simulink model "tesla_model"  (R2017b)
settings: Solver=VariableStepAuto  StartTime=0.0  StopTime=time  RelTol=1e-3
values from neighbouring files (symbols this model uses):
  fd = 0.5*density*A*C_D    (= 0.34398)    [tesla_model.m]
  fr = mass*g*C_r    (= 413.5896)    [tesla_model.m]
  ft = G_r*eta*(1/r)    (= 28.3791666667)    [tesla_model.m]
  G_r = 9.73    [tesla_model.m]
  K_E = 0.12    [tesla_model.m]
  K_T = 0.25    [tesla_model.m]
  L = 493*10^(-9)    (= 4.93e-07)    [tesla_model.m]
  lowLimit = 0    [tesla_model.m]
  mass = 2108    [tesla_model.m]
  r = 0.5*d    (= 0.24)    [tesla_model.m]
  R = 5.3*10^(-3)    (= 0.0053)    [tesla_model.m]
  uppLimit = 601    [tesla_model.m]
  V = mod*groups*v_nom    (= 345.6)    [tesla_model.m]
settings Model: Creator=User1  LastModifiedBy=User1

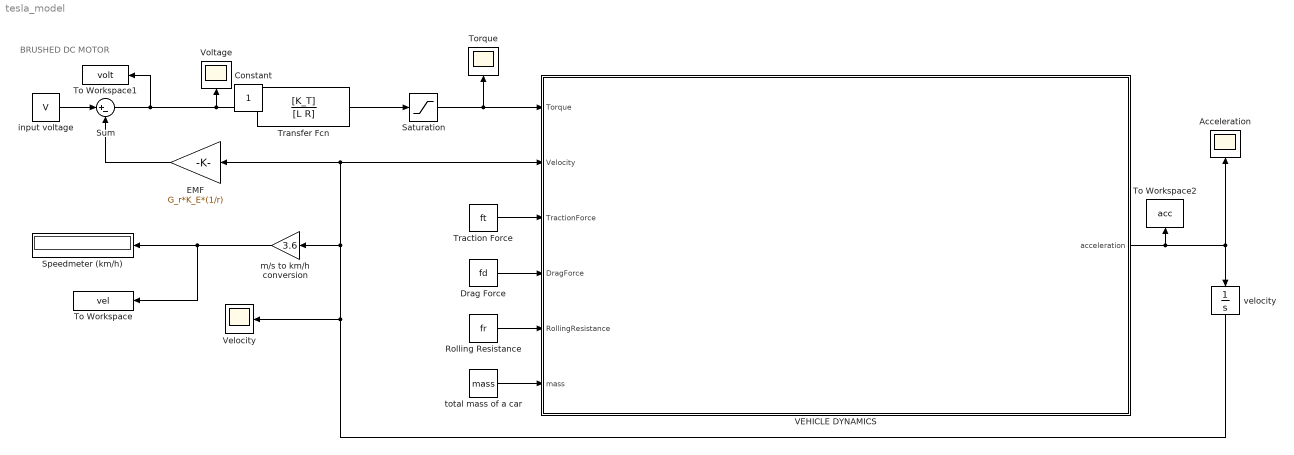
== system tesla_model ==
  note: BRUSHED DC MOTOR
  Acceleration : Scope
  Drag Force : Constant  Value=fd
  EMF : Gain  Gain=G_r*K_E*(1/r)
  Rolling Resistance : Constant  Value=fr
  Saturation : Saturate  UpperLimit=uppLimit  LowerLimit=lowLimit
  Speedmeter (km/h) : Display
  Sum : Sum  Inputs=|+-
  To Workspace : ToWorkspace  VariableName=vel  SaveFormat=Timeseries  SampleTime=-1
      settings: Save2DSignal=2-D array (concatenate along first dimension)
  To Workspace1 : ToWorkspace  VariableName=volt  SaveFormat=Timeseries  SampleTime=-1
      settings: Save2DSignal=2-D array (concatenate along first dimension)
  To Workspace2 : ToWorkspace  VariableName=acc  SaveFormat=Timeseries  SampleTime=-1
  Torque : Scope
  Traction Force : Constant  Value=ft
  Transfer Fcn : TransferFcn  Numerator=[K_T]  Denominator=[L R]
  VEHICLE DYNAMICS : MATLAB Function  TreatAsAtomicUnit=on
  Velocity : Scope
  Voltage : Scope
  input voltage : Constant  Value=V
  m/s to km/h conversion : Gain  Gain=3.6
  total mass of a car : Constant  Value=mass
  velocity : Integrator
  Constant : Constant  IOType=siggen
  wires:
  EMF/1 -> Sum/2
  input voltage/1 -> Sum/1
  Sum/1 -> To Workspace1/1, Transfer Fcn/1, Voltage/1
  Transfer Fcn/1 -> Saturation/1
  velocity/1 -> Velocity/1, m/s to km/h conversion/1, VEHICLE DYNAMICS/2(Velocity), EMF/1
  Drag Force/1 -> VEHICLE DYNAMICS/4(DragForce)
  Rolling Resistance/1 -> VEHICLE DYNAMICS/5(RollingResistance)
  total mass of a car/1 -> VEHICLE DYNAMICS/6(mass)
  Traction Force/1 -> VEHICLE DYNAMICS/3(TractionForce)
  VEHICLE DYNAMICS/1(acceleration) -> To Workspace2/1, velocity/1, Acceleration/1
  m/s to km/h conversion/1 -> To Workspace/1, Speedmeter (km/h)/1
  Saturation/1 -> VEHICLE DYNAMICS/1(Torque), Torque/1

== matlab function tesla_model/VEHICLE DYNAMICS ==
  data: Torque input; acceleration output; Velocity input; TractionForce input; DragForce input; RollingResistance input; mass input
function acceleration = acc(Torque, Velocity, TractionForce, DragForce, RollingResistance, mass)
% Uses 2nd newton law: a = F/m
% acceleration = (Traction Force - Drag Force - Roling Resistance)/mass
acceleration = (Torque*TractionForce-DragForce*Velocity^2-RollingResistance)/mass;
